simulink model "aufgabe_3"  (R2017b)
settings: Solver=VariableStepAuto  StartTime=0.0  StopTime=10.0  RelTol=1e-3
values from neighbouring files (symbols this model uses):
  Cr = ((km*i)-Mm(:,4))./W(:,4)    [aufgabe2_cr.m]    (also in aufgabe3.m = 5e-06; aufgabe4.m = 5e-06; aufgabe6.m = 5e-06)
  i = 0:delta_i:2    [aufgabe1_1.m]    (also in aufgabe2_cr.m = (U0-(ke*W(:,4)))/R)
  J = 0.5e-6    (= 5e-07)    [aufgabe3.m]    (also in aufgabe4.m = 3e-06; aufgabe6.m = 3e-06)
  ke = 0.024    [aufgabe2_cr.m]    (also in aufgabe3.m; aufgabe4.m; aufgabe6.m)
  km = 0.0232    [aufgabe2_cr.m]    (also in aufgabe3.m = 0.0227; aufgabe4.m = 0.023; aufgabe6.m = 0.023)
  L = Lm+Ls    [aufgabe2.m]    (also in aufgabe2_cr.m = 0.0004; aufgabe3.m = 0.0004; aufgabe4.m = 0.0004; aufgabe6.m = 0.0004)
  Ml = 0    [aufgabe2_cr.m]    (also in aufgabe3.m; aufgabe6.m)
  R = 3+(2*rand-1)*0.4    [aufgabe1.m]    (also in aufgabe2.m = 3; aufgabe2_cr.m = 3; aufgabe3.m = 3; aufgabe4.m = 3)
  U0 = 12    [aufgabe2_cr.m]    (also in aufgabe3.m; aufgabe4.m = 20; aufgabe6.m)
undefined symbols (not defined in the file or in its folder): W
settings Model: Creator=gurbuz  LastModifiedBy=gurbuz

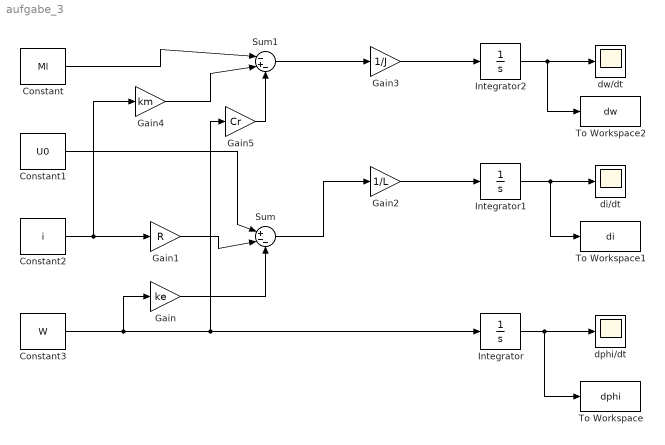
== system aufgabe_3 ==
  Constant : Constant  Value=Ml
  Constant1 : Constant  Value=U0
  Constant2 : Constant  Value=i
  Constant3 : Constant  Value=W
  Gain : Gain  Gain=ke
  Gain1 : Gain  Gain=R
  Gain2 : Gain  Gain=1/L
  Gain3 : Gain  Gain=1/J
  Gain4 : Gain  Gain=km
  Gain5 : Gain  Gain=Cr
  Integrator : Integrator
  Integrator1 : Integrator
  Integrator2 : Integrator
  Sum : Sum  Inputs=|+--
  Sum1 : Sum  Inputs=|-+-
  To Workspace : ToWorkspace  VariableName=dphi  SaveFormat=Timeseries  SampleTime=-1
  To Workspace1 : ToWorkspace  VariableName=di  SaveFormat=Timeseries  SampleTime=-1
  To Workspace2 : ToWorkspace  VariableName=dw  SaveFormat=Timeseries  SampleTime=-1
  "di/dt " : Scope
  "dphi/dt " : Scope
  "dw/dt " : Scope
  wires:
  Constant3/1 -> Gain/1, Gain5/1, Integrator/1
  Integrator/1 -> To Workspace/1, "dphi/dt "/1
  Integrator1/1 -> "di/dt "/1, To Workspace1/1
  Integrator2/1 -> To Workspace2/1, "dw/dt "/1
  Gain/1 -> Sum/3
  Constant2/1 -> Gain4/1, Gain1/1
  Gain1/1 -> Sum/2
  Constant1/1 -> Sum/1
  Sum/1 -> Gain2/1
  Gain2/1 -> Integrator1/1
  Gain3/1 -> Integrator2/1
  Gain4/1 -> Sum1/2
  Constant/1 -> Sum1/1
  Sum1/1 -> Gain3/1
  Gain5/1 -> Sum1/3
